simulink model "parent_test"  (R2025a)
settings: Solver=VariableStepAuto  StartTime=0.0  StopTime=inf  RelTol=1e-3
settings Model: PacingRate=0.500000  Creator=matthewkeller  LastModifiedBy=ryanjing

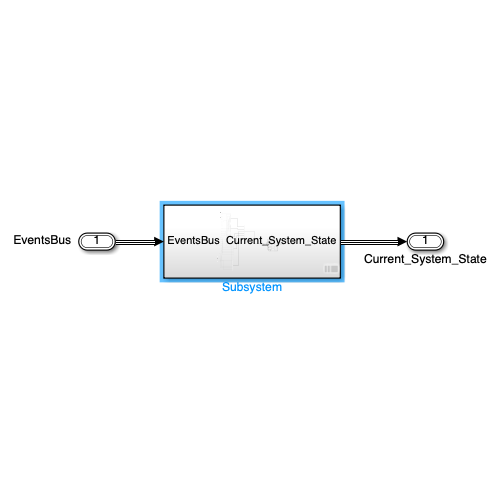
[thumbnail: Simulink's stored preview of the top-level diagram]
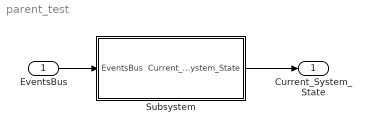
== system parent_test ==
  EventsBus : Inport  OutDataTypeStr=Bus: EventsBus
  Subsystem : Subsystem
  Current_System_State : Outport  OutDataTypeStr=Bus: CurrentStateBus
  wires:
  EventsBus/1 -> Subsystem/1(EventsBus)
  Subsystem/1(Current_System_State) -> Current_System_State/1

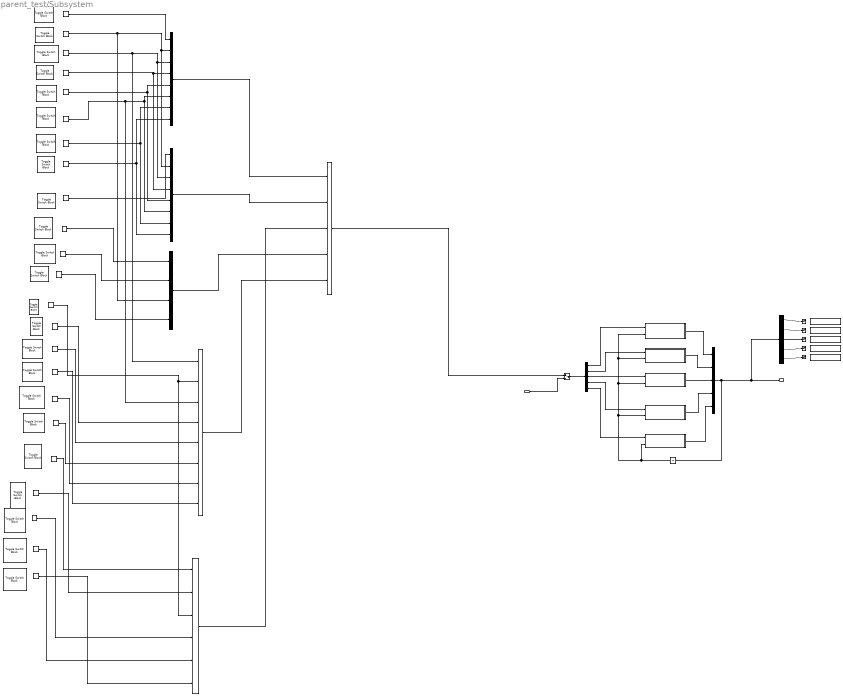
== system parent_test/Subsystem ==
  EventsBus : Inport  OutDataTypeStr=Bus: EventsBus
  ACC_Enable_Pressed : Constant  OutDataTypeStr=boolean
  Activate_AIN_Pressed : Constant  Value=0  OutDataTypeStr=boolean
  Activate_AP_Pressed : Constant  Value=0  OutDataTypeStr=boolean
  Activate_LCC_Pressed : Constant  Value=0  OutDataTypeStr=boolean
  Bus Creator : BusCreator  Inputs=5  OutDataTypeStr=Bus: CurrentStateBus
      settings: InheritFromInputs=off
  Bus Creator1 : BusCreator  Inputs=8  OutDataTypeStr=Bus: ACCStatusBus
  Bus Creator2 : BusCreator  Inputs=8  OutDataTypeStr=Bus: CACCStatusBus
  Bus Creator3 : BusCreator  Inputs=4  OutDataTypeStr=Bus: AINStatusBus
  Bus Creator4 : BusCreator  Inputs=8
  Bus Creator5 : BusCreator  Inputs=6  OutDataTypeStr=Bus: LCCStatusBus
  Bus Creator6 : BusCreator  Inputs=5  OutDataTypeStr=Bus: EventsBus
  Bus Selector : BusSelector  OutputSignals=ACCStatusBus,CACCStatusBus,LCCStatusBus,AINStatusBus,APStatusBus
  Bus Selector1 : BusSelector  OutputSignals=ACCStatus,APStatus,AINStatus,LCCStatus,CACCStatus
  CACC_Enable_Pressed : Constant  Value=0  OutDataTypeStr=boolean
  Cancel_AIN_Pressed : Constant  Value=0  OutDataTypeStr=boolean
  Cancel_AP_Pressed : Constant  Value=0  OutDataTypeStr=boolean
  Cancel_LCC_Pressed : Constant  Value=0  OutDataTypeStr=boolean
  Cancel_Pressed : Constant  Value=0  OutDataTypeStr=boolean
  Display{,1..4} (5 alike) : DisplayBlock  LabelPosition=Hide  Transparency=1  GridColor=[0.502, 0.502, 0.502]
  Driver_Brakes : Constant  Value=0  OutDataTypeStr=boolean
  Driver_Inactivity_Detected : Constant  Value=0  OutDataTypeStr=boolean
  Finish_Pressed : Constant  Value=0  OutDataTypeStr=boolean
  In_CACC_Speed_Range : Constant  Value=0  OutDataTypeStr=boolean
  Is_Stationary : Constant  Value=0  OutDataTypeStr=boolean
  Lane_Change_Centred : Constant  Value=0  OutDataTypeStr=boolean
  Lateral_Switch_ON : Constant  Value=0  OutDataTypeStr=boolean
  Longitudinal_Switch_ON : Constant  Value=0  OutDataTypeStr=boolean
  Manual Switch : ManualSwitch
  Model : ModelReference  ModelNameDialog=acc  SimulationMode=Normal  ModelReferenceVersion=1.53
  Model1 : ModelReference  ModelNameDialog=lcc  SimulationMode=Normal  ModelReferenceVersion=1.39
  Model2 : ModelReference  ModelNameDialog=cacc  SimulationMode=Normal  ModelReferenceVersion=1.51
  Model3 : ModelReference  ModelNameDialog=ain  SimulationMode=Normal  ModelReferenceVersion=1.47
  Model4 : ModelReference  ModelNameDialog=ap  SimulationMode=Normal  ModelReferenceVersion=1.39
  Parking_In_Range : Constant  Value=0  OutDataTypeStr=boolean
  Set_Resume : Constant  Value=0  OutDataTypeStr=boolean
  Speed_GT_35_MPH : Constant  Value=0  OutDataTypeStr=boolean
  Speed_LT_55_MPH : Constant  Value=0  OutDataTypeStr=boolean
  Terminator{,1..4} (5 alike) : Terminator
  Timeout_Event : Constant  Value=0  OutDataTypeStr=boolean
  Toggle Switch{,1..22} (23 alike) : ToggleSwitchBlock
  Unit Delay : UnitDelay  SampleTime=-1  HasFrameUpgradeWarning=on
  V2X_Switch_ON : Constant  Value=0  OutDataTypeStr=boolean
  Current_System_State : Outport
  wires:
  Bus Selector/4 -> Model3/1  "<AINStatusBus>"
  Bus Selector/3 -> Model1/1  "<LCCStatusBus>"
  Bus Selector/1 -> Model/1  "<ACCStatusBus>"
  Bus Selector/2 -> Model2/1  "<CACCStatusBus>"
  Bus Selector/5 -> Model4/1  "<APStatusBus>"
  EventsBus/1 -> Manual Switch/2  "EventsBus"
  Bus Creator/1 -> Bus Selector1/1, Current_System_State/1, Unit Delay/1
  Model/1 -> Bus Creator/1
  Model2/1 -> Bus Creator/2
  Model1/1 -> Bus Creator/3
  Model3/1 -> Bus Creator/4
  Model4/1 -> Bus Creator/5
  Unit Delay/1 -> Model3/2, Model/2, Model2/2, Model1/2, Model4/2
  Activate_LCC_Pressed/1 -> Bus Creator5/4  "Activate_LCC_Pressed"
  Speed_GT_35_MPH/1 -> Bus Creator5/2  "Speed_GT_35_MPH"
  Bus Creator6/1 -> Manual Switch/1
  Set_Resume/1 -> Bus Creator2/4, Bus Creator1/4  "Set_Resume"
  Is_Stationary/1 -> Bus Creator4/4  "Is_Stationary"
  V2X_Switch_ON/1 -> Bus Creator3/3, Bus Creator2/2, Bus Creator1/2  "V2X_Switch_ON"
  Timeout_Event/1 -> Bus Creator1/7, Bus Creator2/7  "Timeout_Event"
  Bus Creator3/1 -> Bus Creator6/4  "AINStatusBus"
  Activate_AP_Pressed/1 -> Bus Creator4/5  "Activate_AP_Pressed"
  In_CACC_Speed_Range/1 -> Bus Creator2/8, Bus Creator1/8  "In_CACC_Speed_Range"
  Driver_Inactivity_Detected/1 -> Bus Creator5/6  "Driver_Inactivity_Detected"
  Bus Creator2/1 -> Bus Creator6/2  "CACCStatusBus"
  Activate_AIN_Pressed/1 -> Bus Creator3/1  "Activate_AIN_Pressed"
  Bus Creator1/1 -> Bus Creator6/1  "ACCStatusBus"
  Lane_Change_Centred/1 -> Bus Creator5/1  "Lane_Change_Centred"
  CACC_Enable_Pressed/1 -> Bus Creator2/1  "CACC_Enable_Pressed"
  Cancel_LCC_Pressed/1 -> Bus Creator5/5  "Cancel_LCC_Pressed"
  Cancel_AIN_Pressed/1 -> Bus Creator3/2  "Cancel_AIN_Pressed"
  Lateral_Switch_ON/1 -> Bus Creator5/3, Bus Creator4/2  "Lateral_Switch_ON"
  ACC_Enable_Pressed/1 -> Bus Creator1/1  "ACC_Enable_Pressed"
  Cancel_Pressed/1 -> Bus Creator1/5, Bus Creator2/5  "Cancel_Pressed"
  Finish_Pressed/1 -> Bus Creator4/7  "Finish_Pressed"
  Cancel_AP_Pressed/1 -> Bus Creator4/8  "Cancel_AP_Pressed"
  Longitudinal_Switch_ON/1 -> Bus Creator4/1, Bus Creator2/3, Bus Creator1/3  "Longitudinal_Switch_ON"
  Bus Creator5/1 -> Bus Creator6/3  "LCCStatusBus"
  Parking_In_Range/1 -> Bus Creator4/6  "Parking_In_Range"
  Bus Creator4/1 -> Bus Creator6/5  "APStatusBus"
  Speed_LT_55_MPH/1 -> Bus Creator3/4  "Speed_LT_55_MPH"
  Driver_Brakes/1 -> Bus Creator4/3, Bus Creator1/6, Bus Creator2/6  "Driver_Brakes"
  Manual Switch/1 -> Bus Selector/1
  Bus Selector1/1 -> Terminator/1  "<ACCStatus>"
  Bus Selector1/2 -> Terminator1/1  "<APStatus>"
  Bus Selector1/3 -> Terminator2/1  "<AINStatus>"
  Bus Selector1/4 -> Terminator3/1  "<LCCStatus>"
  Bus Selector1/5 -> Terminator4/1  "<CACCStatus>"
